simulink model "gate"  (R2025b)
settings: Solver=FixedStepAuto  StartTime=0.0  StopTime=10.0  FixedStep=Ts_local  RelTol=1e-3
model workspace (MAT data in the model file):
  Ksvl = 0.0276
  Ksvr = 0.04
  Xmax = 0.006
  Xmin = -0.004
  dl = -0.014
  dr = 0.014
  k = 0.15
libraries: simulink x2
settings Model: DataDictionary=ctrlSys.sldd  ParameterArgumentNames=Ksvl,Ksvr,Xmax,Xmin,dl,dr,k  Creator=LYG  LastModifiedBy=LYG

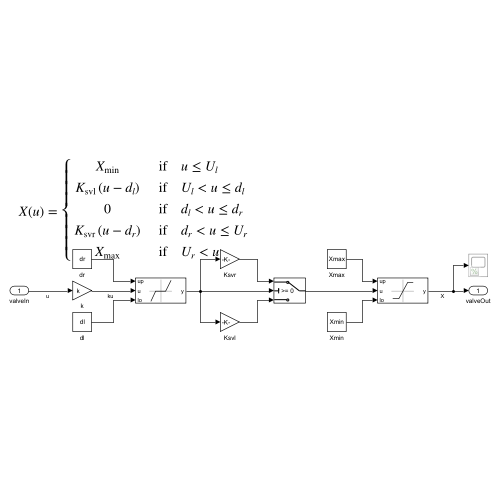
[thumbnail: Simulink's stored preview of the top-level diagram]
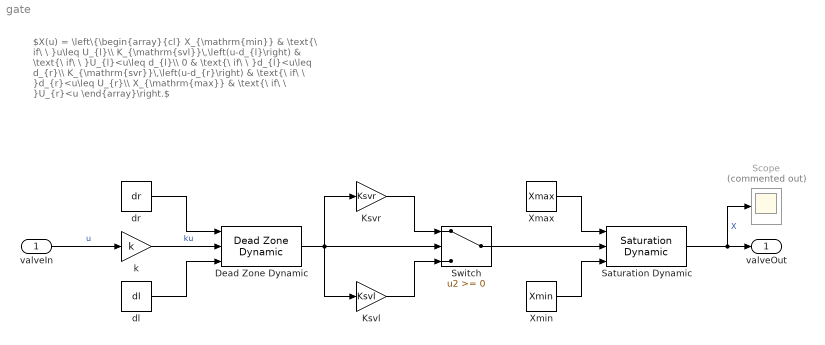
== system gate ==
  note: $X(u) = \left\{\begin{array}{cl} X_{\mathrm{min}} & \text{\ if\ \ }u\leq U_{l}\\ K_{\mathrm{svl}}\,\left(u-d_{l}\right) & \text{\ if\ \ }U_{l}<u\leq d_{l}\\ 0 & \text{\ if\ \ }d_{l}<u\leq d_{r}\\ K_{\mathrm{svr}}\,\left(u-d_{r}\right) & \text{\ if\ \ }d_{r}<u\leq U_{r}\\ X_{\mathrm{max}} & \text{\ if\ \ }U_{r}<u \end{array}\right.$
  valveIn : Inport
  Dead Zone Dynamic : simulink/Discontinuities/Dead Zone Dynamic
  Ksvl : Gain  Gain=Ksvl
  Ksvr : Gain  Gain=Ksvr
  Saturation Dynamic : simulink/Discontinuities/Saturation Dynamic  OutMin=[]  OutMax=[]  OutDataTypeStr=Inherit: Same as second input  OutDataType=fixdt(1, 16)  OutScaling=2^-10  DoSatur=off
  Scope : Scope  Commented=on
      settings: ActiveDisplayYMinimum=-0.18694  ActiveDisplayYMaximum=0.18694
  Switch : Switch  SaturateOnIntegerOverflow=off  InputSameDT=off
  Xmax : Constant  Value=Xmax
  Xmin : Constant  Value=Xmin
  dl : Constant  Value=dl
  dr : Constant  Value=dr
  k : Gain  Gain=k
  valveOut : Outport
  wires:
  valveIn/1 -> k/1  "u"
  dr/1 -> Dead Zone Dynamic/1
  dl/1 -> Dead Zone Dynamic/3
  Xmax/1 -> Saturation Dynamic/1
  Xmin/1 -> Saturation Dynamic/3
  Dead Zone Dynamic/1 -> Ksvl/1, Ksvr/1, Switch/2
  Ksvr/1 -> Switch/1
  Ksvl/1 -> Switch/3
  k/1 -> Dead Zone Dynamic/2  "ku"
  Switch/1 -> Saturation Dynamic/2
  Saturation Dynamic/1 -> Scope/1, valveOut/1  "X"
